simulink model "Tadpole_throttlecontroller_mockup"  (R2023b)
settings: Solver=VariableStepAuto  StartTime=0.0  StopTime=10.0  RelTol=1e-3
settings Model: Creator=Andrew Radulovich  LastModifiedBy=Andrew Radulovich

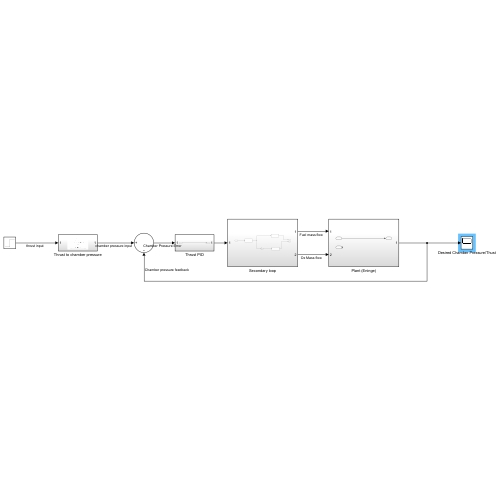
[thumbnail: Simulink's stored preview of the top-level diagram]
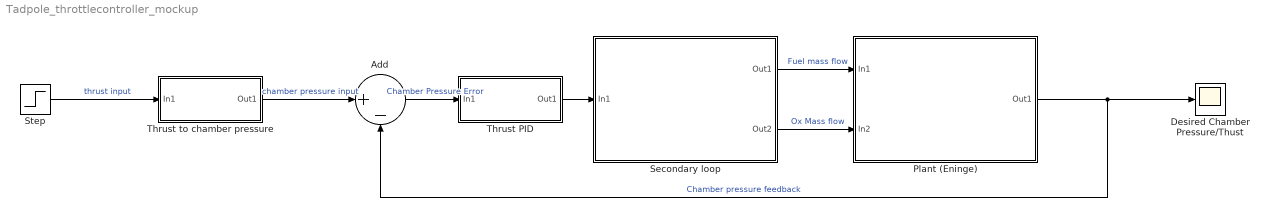
== system Tadpole_throttlecontroller_mockup ==
  Add : Sum  Inputs=|+-
  Desired Chamber Pressure/Thust : Scope
  Plant (Eninge) : Subsystem
  Secondary loop : Subsystem
  Step : Step  SampleTime=0
  Thrust PID : Subsystem
  Thrust to chamber pressure : Subsystem
  wires:
  Step/1 -> Thrust to chamber pressure/1(In1)  "thrust input"
  Thrust to chamber pressure/1(Out1) -> Add/1  "chamber pressure input"
  Plant (Eninge)/1(Out1) -> Desired Chamber Pressure/Thust/1, Add/2  "Chamber pressure feedback"
  Add/1 -> Thrust PID/1(In1)  "Chamber Pressure Error"
  Thrust PID/1(Out1) -> Secondary loop/1(In1)
  Secondary loop/1(Out1) -> Plant (Eninge)/1(In1)  "Fuel mass flow"
  Secondary loop/2(Out2) -> Plant (Eninge)/2(In2)  "Ox Mass flow"

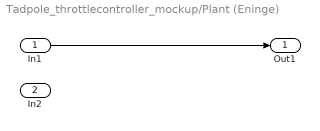
== system Tadpole_throttlecontroller_mockup/Plant (Eninge) ==
  In1 : Inport
  In2 : Inport  Port=2
  Out1 : Outport
  wires:
  In1/1 -> Out1/1

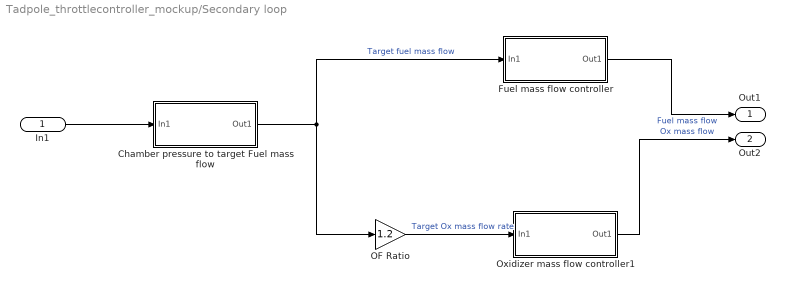
== system Tadpole_throttlecontroller_mockup/Secondary loop ==
  In1 : Inport
  Chamber pressure to target Fuel mass flow : Subsystem
  Fuel mass flow controller : Subsystem
  OF Ratio : Gain  Gain=1.2
  Oxidizer mass flow controller1 : Subsystem
  Out1 : Outport
  Out2 : Outport  Port=2
  wires:
  In1/1 -> Chamber pressure to target Fuel mass flow/1(In1)
  Chamber pressure to target Fuel mass flow/1(Out1) -> OF Ratio/1, Fuel mass flow controller/1(In1)  "Target fuel mass flow"
  OF Ratio/1 -> Oxidizer mass flow controller1/1(In1)  "Target Ox mass flow rate"
  Fuel mass flow controller/1(Out1) -> Out1/1  "Fuel mass flow"
  Oxidizer mass flow controller1/1(Out1) -> Out2/1  "Ox mass flow"

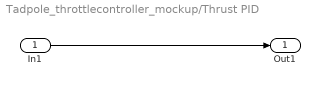
== system Tadpole_throttlecontroller_mockup/Thrust PID ==
  In1 : Inport
  Out1 : Outport
  wires:
  In1/1 -> Out1/1

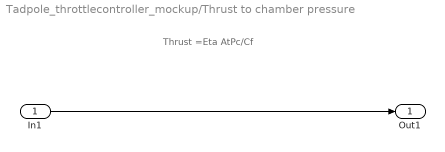
== system Tadpole_throttlecontroller_mockup/Thrust to chamber pressure ==
  note: Thrust =Eta AtPc/Cf
  In1 : Inport
  Out1 : Outport
  wires:
  In1/1 -> Out1/1

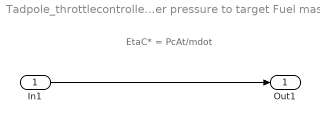
== system Tadpole_throttlecontroller_mockup/Secondary loop/Chamber pressure to target Fuel mass flow ==
  note: EtaC* = PcAt/mdot
  In1 : Inport
  Out1 : Outport
  wires:
  In1/1 -> Out1/1

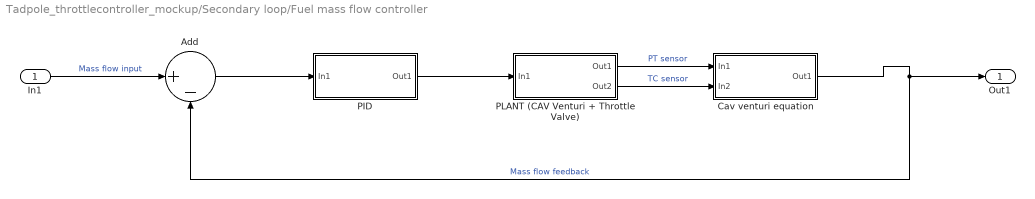
== system Tadpole_throttlecontroller_mockup/Secondary loop/Fuel mass flow controller ==
  In1 : Inport
  Add : Sum  Inputs=|+-
  Cav venturi equation : Subsystem
  PID : Subsystem
  PLANT (CAV Venturi + Throttle Valve) : Subsystem
  Out1 : Outport
  wires:
  In1/1 -> Add/1  "Mass flow input"
  Add/1 -> PID/1(In1)
  PID/1(Out1) -> PLANT (CAV Venturi + Throttle Valve)/1(In1)
  PLANT (CAV Venturi + Throttle Valve)/1(Out1) -> Cav venturi equation/1(In1)  "PT sensor"
  PLANT (CAV Venturi + Throttle Valve)/2(Out2) -> Cav venturi equation/2(In2)  "TC sensor"
  Cav venturi equation/1(Out1) -> Add/2, Out1/1  "Mass flow feedback"

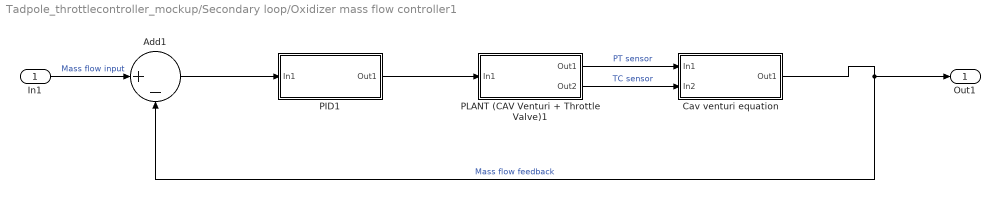
== system Tadpole_throttlecontroller_mockup/Secondary loop/Oxidizer mass flow controller1 ==
  In1 : Inport
  Add1 : Sum  Inputs=|+-
  Cav venturi equation : Subsystem
  PID1 : Subsystem
  PLANT (CAV Venturi + Throttle Valve)1 : Subsystem
  Out1 : Outport
  wires:
  Cav venturi equation/1(Out1) -> Add1/2, Out1/1  "Mass flow feedback"
  PID1/1(Out1) -> PLANT (CAV Venturi + Throttle Valve)1/1(In1)
  PLANT (CAV Venturi + Throttle Valve)1/2(Out2) -> Cav venturi equation/2(In2)  "TC sensor"
  Add1/1 -> PID1/1(In1)
  PLANT (CAV Venturi + Throttle Valve)1/1(Out1) -> Cav venturi equation/1(In1)  "PT sensor"
  In1/1 -> Add1/1  "Mass flow input"

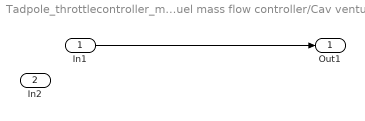
== system Tadpole_throttlecontroller_mockup/Secondary loop/Fuel mass flow controller/Cav venturi equation ==
  In1 : Inport
  In2 : Inport  Port=2
  Out1 : Outport
  wires:
  In1/1 -> Out1/1

== system Tadpole_throttlecontroller_mockup/Secondary loop/Fuel mass flow controller/PID ==
  In1 : Inport
  Out1 : Outport
  wires:
  In1/1 -> Out1/1

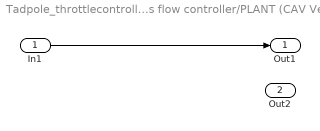
== system Tadpole_throttlecontroller_mockup/Secondary loop/Fuel mass flow controller/PLANT (CAV Venturi + Throttle Valve) ==
  In1 : Inport
  Out1 : Outport
  Out2 : Outport  Port=2
  wires:
  In1/1 -> Out1/1

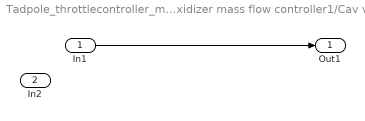
== system Tadpole_throttlecontroller_mockup/Secondary loop/Oxidizer mass flow controller1/Cav venturi equation ==
  In1 : Inport
  In2 : Inport  Port=2
  Out1 : Outport
  wires:
  In1/1 -> Out1/1

== system Tadpole_throttlecontroller_mockup/Secondary loop/Oxidizer mass flow controller1/PID1 ==
  In1 : Inport
  Out1 : Outport
  wires:
  In1/1 -> Out1/1

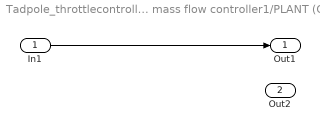
== system Tadpole_throttlecontroller_mockup/Secondary loop/Oxidizer mass flow controller1/PLANT (CAV Venturi + Throttle Valve)1 ==
  In1 : Inport
  Out1 : Outport
  Out2 : Outport  Port=2
  wires:
  In1/1 -> Out1/1
